simulink model "MatTransEx"  (R2015a)
settings: Solver=FixedStepDiscrete  StartTime=0.0  StopTime=tsim  FixedStep=dt  RelTol=1e-3
values from neighbouring files (symbols this model uses):
  Cp1d = Cp1*ones(length(y0),1)'    [run_MatTransEx.m]
  Cp2d = Cp1*ones(length(y0),length(x))    [run_MatTransEx.m]
  hb = 0.05    [run_MatTransEx.m]
  hl = 0.05    [run_MatTransEx.m]
  hr = 0.05    [run_MatTransEx.m]
  ht = 0.05    [run_MatTransEx.m]
  k1d = k1*ones(length(y0),1)'    [run_MatTransEx.m]
  k2d = k1*ones(length(y0),length(x))    [run_MatTransEx.m]
  m = length(y0)    [run_MatTransEx.m]
  n = length(x)    [run_MatTransEx.m]
  rho1d = rho1*ones(length(y0),1)'    [run_MatTransEx.m]
  rho2d = rho1*ones(length(y0),length(x))    [run_MatTransEx.m]
  Tb = 650    [run_MatTransEx.m]
  Tl = 650    [run_MatTransEx.m]
  Tr = 550    [run_MatTransEx.m]
  Tt = 550    [run_MatTransEx.m]
libraries: lib_Conduction_HeatX1DVarPropsAndGenBCs x1, lib_Conduction_2DCondFullyImplicit x1
settings Model: Creator=jlkratz  LastModifiedBy=jlkratz

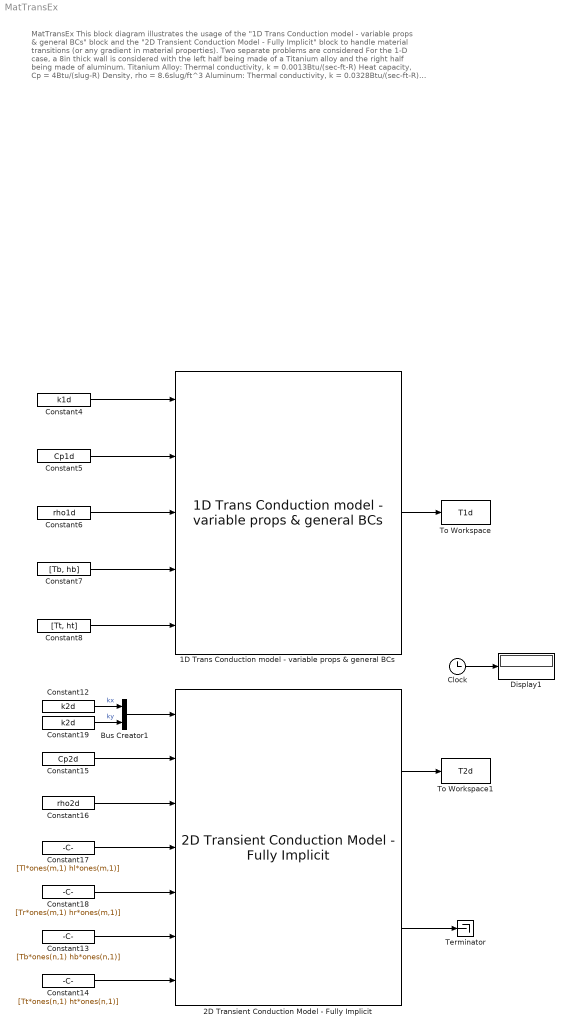
== system MatTransEx ==
  note: MatTransEx
      |
      | This block diagram illustrates the usage of the "1D Trans Conduction model - variable props & general BCs" block and
      | the "2D Transient Conduction Model - Fully Implicit" block to handle material transitions (or any gradient in
      | material properties). Two separate problems are considered
      |
      | For the 1-D case, a 8in thick wall is considered with the left half being made of a Titanium alloy and the right half being
      | made of aluminum.
      | Titanium Alloy:
      | Thermal conductivity, k = 0.0013Btu/(sec-ft-R)
      | Heat capacity, Cp = 4Btu/(slug-R)
      | Density, rho = 8.6slug/ft^3
      | Aluminum:
      | Thermal conductivity, k = 0.0328Btu/(sec-ft-R)
      | Heat capacity, Cp = 6.92Btu/(slug-R)
      | Density, rho = 5.24slug/ft^3
      | The entire structure starts at 550R. The wall is heated on the left side by convection with a fluid temperature of 650R and
      | a heat transfer coefficient of 0.05Btu/(sec-ft^2-R).
      |
      | For the 2-D case, an 8in by 8in bar is considered with the bottom left quadrant being made of the Titanium alloy and the
      | rest being made of aluminum. The boundary conditions are as follows:
      | Bottom: Temperature = 650R, Heat Transfer Coefficient = 0.05Btu/(sec-ft^2-R)
      | Top: Temperature = 550R, Heat Transfer Coefficient = 0.05Btu/(sec-ft^2-R)
      | Left: Temperature = 650R, Heat Transfer Coefficient = 0.05Btu/(sec-ft^2-R)
      | Right: Temperature = 550R, Heat Transfer Coefficient = 0.05Btu/(sec-ft^2-R)
  1D Trans Conduction model - variable props & general BCs : lib_Conduction_HeatX1DVarPropsAndGenBCs/1D Trans Conduction model - variable props & general BCs  x_M=y0  T0_M=T01d  dt_M=dt  a_M=off  convin_M=on  radin_M=off  condin_M=off  convout_M=on  radout_M=off  condout_M=off  BN_M=double(gcb)
  2D Transient Conduction Model - Fully Implicit : lib_Conduction_2DCondFullyImplicit/2D Transient Conduction Model - Fully Implicit  T0_M=T02d  dt_M=dt  x_M=x  y_M=y0  shape_M=Planar in both directions  convL_M=on  radL_M=off  condL_M=off  convR_M=on  radR_M=off  condR_M=off  convB_M=on  radB_M=off  condB_M=off  convT_M=on  radT_M=off  condT_M=off  BN_M=double(gcb)
  Bus Creator1 : BusCreator  Inputs=2
  Clock : Clock
  Constant12 : Constant  Value=k2d
  Constant13 : Constant  Value=[Tb*ones(n,1) hb*ones(n,1)]
  Constant14 : Constant  Value=[Tt*ones(n,1) ht*ones(n,1)]
  Constant15 : Constant  Value=Cp2d
  Constant16 : Constant  Value=rho2d
  Constant17 : Constant  Value=[Tl*ones(m,1) hl*ones(m,1)]
  Constant18 : Constant  Value=[Tr*ones(m,1) hr*ones(m,1)]
  Constant19 : Constant  Value=k2d
  Constant4 : Constant  Value=k1d
  Constant5 : Constant  Value=Cp1d
  Constant6 : Constant  Value=rho1d
  Constant7 : Constant  Value=[Tb, hb]
  Constant8 : Constant  Value=[Tt, ht]
  Display1 : Display
  Terminator : Terminator
  To Workspace : ToWorkspace  VariableName=T1d  SaveFormat=Timeseries  SampleTime=-1
  To Workspace1 : ToWorkspace  VariableName=T2d  SaveFormat=Timeseries  SampleTime=-1
  wires:
  Constant4/1 -> 1D Trans Conduction model - variable props & general BCs/1
  Constant5/1 -> 1D Trans Conduction model - variable props & general BCs/2
  Constant6/1 -> 1D Trans Conduction model - variable props & general BCs/3
  Constant7/1 -> 1D Trans Conduction model - variable props & general BCs/4
  Constant8/1 -> 1D Trans Conduction model - variable props & general BCs/5
  1D Trans Conduction model - variable props & general BCs/1 -> To Workspace/1
  2D Transient Conduction Model - Fully Implicit/1 -> To Workspace1/1
  2D Transient Conduction Model - Fully Implicit/2 -> Terminator/1
  Clock/1 -> Display1/1
  Constant12/1 -> Bus Creator1/1  "kx"
  Constant19/1 -> Bus Creator1/2  "ky"
  Bus Creator1/1 -> 2D Transient Conduction Model - Fully Implicit/1
  Constant15/1 -> 2D Transient Conduction Model - Fully Implicit/2
  Constant16/1 -> 2D Transient Conduction Model - Fully Implicit/3
  Constant14/1 -> 2D Transient Conduction Model - Fully Implicit/7
  Constant13/1 -> 2D Transient Conduction Model - Fully Implicit/6
  Constant17/1 -> 2D Transient Conduction Model - Fully Implicit/4
  Constant18/1 -> 2D Transient Conduction Model - Fully Implicit/5
